simulink model "RRR_ADbst"  (R2022a)
settings: Solver=VariableStepAuto  StartTime=0.0  StopTime=500  RelTol=1e-6
undefined symbols (not defined in the file): DiscIntNeverNeededParam, dq0, Ks_ADbs, Lambda_ADbs, Levenberg, m1, m2, m3, Marquardt, p0, param, Pi, Pi_hat0_ADbs, q0, r0, r1, r2, R_ADbs, slow
libraries: simulink x1, robotmaniplib x1
settings Model: PauseTimes=0.14  Creator=Mathew  LastModifiedBy=Marco
settings SolverCC: ZeroCrossControl=DisableAll  ODENIntegrationMethod=ode1be
settings DebuggingCC: AlgebraicLoopMsg=none  UnconnectedInputMsg=warning  UnconnectedOutputMsg=warning  UnconnectedLineMsg=warning  SFMachineParentedDataDiag=warning
settings SFSimCC: CustomCodeUndefinedFunction=UseInterfaceOnly
settings RTWCC: DLArmComputeVersion=19.05

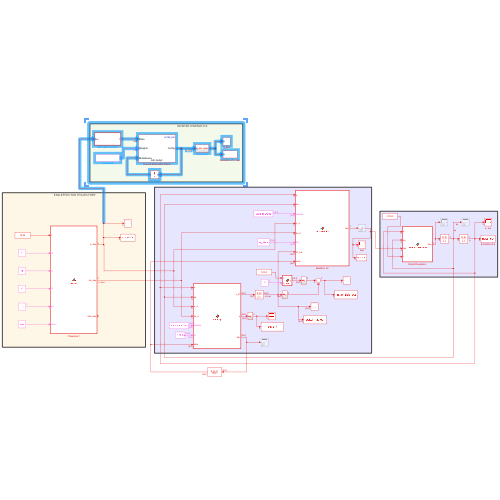
[thumbnail: Simulink's stored preview of the top-level diagram]
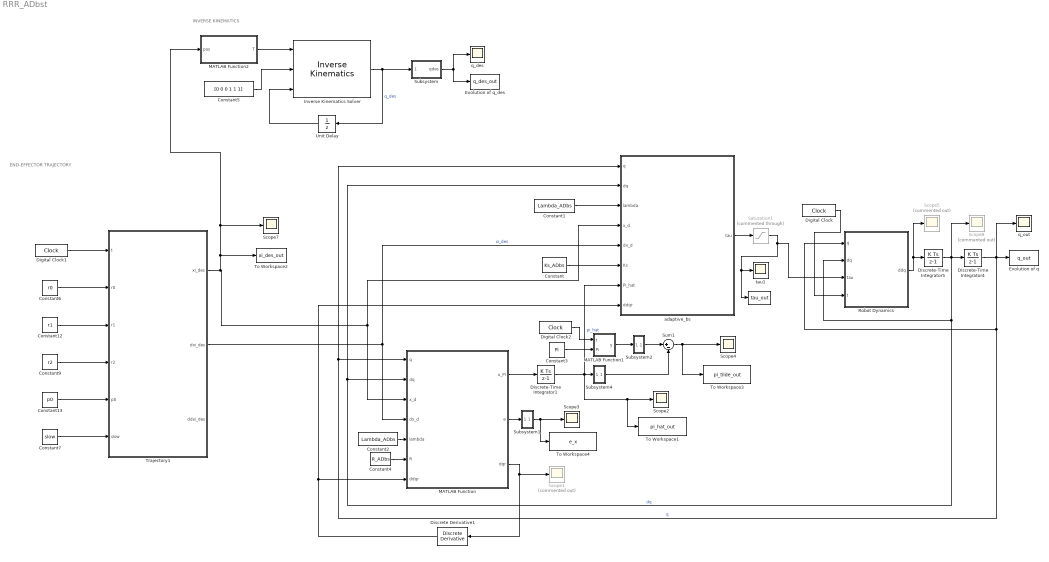
== system RRR_ADbst ==
  note: END-EFFECTOR TRAJECTORY
  note: INVERSE KINEMATICS
  "         " : ToWorkspace  VariableName=tau_out  SaveFormat=Timeseries  SampleTime=-1
  Constant : Constant  Value=Ks_ADbs
  Constant1 : Constant  Value=Lambda_ADbs
  Constant12 : Constant  Value=r1
  Constant13 : Constant  Value=p0
  Constant2 : Constant  Value=Lambda_ADbs
  Constant3 : Constant  Value=Pi
  Constant4 : Constant  Value=R_ADbs
  Constant5 : Constant  Value=[0 0 0 1 1 1]
  Constant6 : Constant  Value=r0
  Constant7 : Constant  Value=slow
  Constant9 : Constant  Value=r2
  Digital Clock : DigitalClock  SampleTime=0.01
  Digital Clock1 : DigitalClock  SampleTime=0.01
  Digital Clock2 : DigitalClock  SampleTime=0.01
  Discrete Derivative1 : simulink/Discrete/Discrete Derivative  gainval=1.0  ICPrevScaledInput=ddq0  OutMin=[]  OutMax=[]  OutDataType=fixdt(1, 16)  OutScaling=2^-10  DoSatur=off
  Discrete-Time Integrator1 : DiscreteIntegrator  InitialCondition=Pi_hat0_ADbs  SampleTime=-1  ICPrevOutput=DiscIntNeverNeededParam  ICPrevScaledInput=DiscIntNeverNeededParam
  Discrete-Time Integrator4 : DiscreteIntegrator  InitialCondition=q0  SampleTime=-1  ICPrevOutput=DiscIntNeverNeededParam  ICPrevScaledInput=DiscIntNeverNeededParam
  Discrete-Time Integrator5 : DiscreteIntegrator  InitialCondition=dq0  SampleTime=-1  ICPrevOutput=DiscIntNeverNeededParam  ICPrevScaledInput=DiscIntNeverNeededParam
  Evolution of q : ToWorkspace  VariableName=q_out  SaveFormat=Timeseries  SampleTime=-1
  Evolution of q_des : ToWorkspace  VariableName=q_des_out  SaveFormat=Timeseries  SampleTime=-1
  Inverse Kinematics Solver : robotmaniplib/Inverse Kinematics  RigidBodyTree=ur10e_bis  EndEffector=body3  ShowInfo=off  SolverName=Levenberg-Marquardt  EnforceJointLimits=on  MaxIterations=1500  MaxTime=10  GradientTolerance=1e-7  SolutionTolerance=1e-5  StepTolerance=1e-14  ErrorChangeTolerance=1e-8  UseErrorDamping=on  DampingBias=0.0025  SimulateUsing=Interpreted execution
  MATLAB Function : MATLAB Function  TreatAsAtomicUnit=on
  MATLAB Function1 : MATLAB Function  TreatAsAtomicUnit=on
  MATLAB Function2 : MATLAB Function  TreatAsAtomicUnit=on
  Robot Dynamics : MATLAB Function  TreatAsAtomicUnit=on
  Saturation1 : Saturate  Commented=through  UpperLimit=100  LowerLimit=-100
  Scope1 : Scope  Commented=on
  Scope{2..4,7} (4 alike) : Scope
  Scope5 : Scope  Commented=on
  Scope8 : Scope  Commented=on
  Subsystem : Subsystem
  Subsystem1 : Subsystem
  Subsystem2 : Subsystem
  Subsystem4 : Subsystem
  Sum1 : Sum  Inputs=|+-
  To Workspace1 : ToWorkspace  VariableName=pi_hat_out  SaveFormat=Timeseries  SampleTime=-1
  To Workspace2 : ToWorkspace  VariableName=xi_des_out  SaveFormat=Timeseries  SampleTime=-1
  To Workspace3 : ToWorkspace  VariableName=pi_tilde_out  SaveFormat=Timeseries  SampleTime=-1
  To Workspace4 : ToWorkspace  VariableName=e_x  SaveFormat=Timeseries  SampleTime=-1
  Trajectory1 : MATLAB Function  TreatAsAtomicUnit=on
  Unit Delay : UnitDelay  SampleTime=-1  HasFrameUpgradeWarning=on
  adaptive_bs : MATLAB Function  TreatAsAtomicUnit=on
  q_des : Scope
  q_out : Scope
  tau1 : Scope
  wires:
  Constant/1 -> adaptive_bs/6(Ks)
  adaptive_bs/1(tau) -> Saturation1/1
  MATLAB Function/1(u_Pi) -> Discrete-Time Integrator1/1
  Sum1/1 -> To Workspace3/1, Scope4/1
  Discrete-Time Integrator1/1 -> To Workspace1/1, Scope2/1, Subsystem4/1(eq), adaptive_bs/7(Pi_hat)  "pi_hat"
  Constant4/1 -> MATLAB Function/6(R)
  Constant2/1 -> MATLAB Function/5(lambda)
  Constant1/1 -> adaptive_bs/3(lambda)
  MATLAB Function/3(dqr) -> Discrete Derivative1/1, Scope1/1
  MATLAB Function/2(e) -> Subsystem1/1(eq)
  Digital Clock/1 -> Robot Dynamics/4(t)
  Discrete-Time Integrator5/1 -> Scope8/1, adaptive_bs/2(dq), MATLAB Function/2(dq), Robot Dynamics/2(dq), Discrete-Time Integrator4/1  "dq"
  Discrete-Time Integrator4/1 -> Evolution of q/1, adaptive_bs/1(q), MATLAB Function/1(q), Robot Dynamics/1(q), q_out/1  "q"
  Robot Dynamics/1(ddq) -> Scope5/1, Discrete-Time Integrator5/1
  Inverse Kinematics Solver/1 -> Subsystem/1(q_des), Unit Delay/1  "q_des"
  Subsystem/1(qdes) -> Evolution of q_des/1, q_des/1
  Saturation1/1 -> "         "/1, tau1/1, Robot Dynamics/3(tau)
  Trajectory1/1(xi_des) -> adaptive_bs/4(x_d), MATLAB Function/3(x_d), MATLAB Function2/1(pos), Scope7/1, To Workspace2/1
  Subsystem4/1(eq_) -> Sum1/2
  Subsystem1/1(eq_) -> To Workspace4/1, Scope3/1
  Trajectory1/2(dxi_des) -> adaptive_bs/5(dx_d), MATLAB Function/4(dx_d)  "xi_des"
  Constant13/1 -> Trajectory1/5(p0)
  Constant7/1 -> Trajectory1/6(slow)
  Constant9/1 -> Trajectory1/4(r2)
  Constant12/1 -> Trajectory1/3(r1)
  Constant5/1 -> Inverse Kinematics Solver/2
  MATLAB Function2/1(T) -> Inverse Kinematics Solver/1
  Unit Delay/1 -> Inverse Kinematics Solver/3
  Digital Clock1/1 -> Trajectory1/1(t)
  Constant6/1 -> Trajectory1/2(r0)
  MATLAB Function1/1(y) -> Subsystem2/1(eq)
  Constant3/1 -> MATLAB Function1/2(Pi)
  Digital Clock2/1 -> MATLAB Function1/1(t)
  Subsystem2/1(eq_) -> Sum1/1
  Discrete Derivative1/1 -> MATLAB Function/7(ddqr), adaptive_bs/8(ddqr)

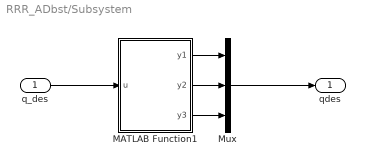
== system RRR_ADbst/Subsystem ==
  q_des : Inport
  MATLAB Function1 : MATLAB Function  TreatAsAtomicUnit=on
  Mux : Mux  Inputs=3
  qdes : Outport
  wires:
  MATLAB Function1/3(y3) -> Mux/3
  MATLAB Function1/2(y2) -> Mux/2
  q_des/1 -> MATLAB Function1/1(u)
  Mux/1 -> qdes/1
  MATLAB Function1/1(y1) -> Mux/1

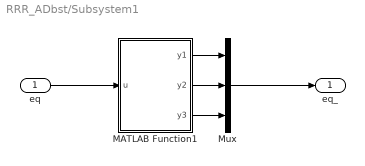
== system RRR_ADbst/Subsystem1 ==
  eq : Inport
  MATLAB Function1 : MATLAB Function  TreatAsAtomicUnit=on
  Mux : Mux  Inputs=3
  eq_ : Outport
  wires:
  MATLAB Function1/3(y3) -> Mux/3
  MATLAB Function1/2(y2) -> Mux/2
  eq/1 -> MATLAB Function1/1(u)
  Mux/1 -> eq_/1
  MATLAB Function1/1(y1) -> Mux/1

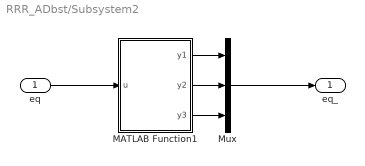
== system RRR_ADbst/Subsystem2 ==
  eq : Inport
  MATLAB Function1 : MATLAB Function  TreatAsAtomicUnit=on
  Mux : Mux  Inputs=3
  eq_ : Outport
  wires:
  MATLAB Function1/1(y1) -> Mux/1
  Mux/1 -> eq_/1
  eq/1 -> MATLAB Function1/1(u)
  MATLAB Function1/2(y2) -> Mux/2
  MATLAB Function1/3(y3) -> Mux/3

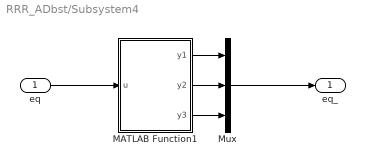
== system RRR_ADbst/Subsystem4 ==
  eq : Inport
  MATLAB Function1 : MATLAB Function  TreatAsAtomicUnit=on
  Mux : Mux  Inputs=3
  eq_ : Outport
  wires:
  MATLAB Function1/1(y1) -> Mux/1
  Mux/1 -> eq_/1
  eq/1 -> MATLAB Function1/1(u)
  MATLAB Function1/2(y2) -> Mux/2
  MATLAB Function1/3(y3) -> Mux/3

== matlab function RRR_ADbst/MATLAB Function1 ==
  data: t input; Pi input; y output
function y = fcn(t,Pi)

    if t > 200
        Pi(2) = Pi(2) + 1;
    end

    y = Pi;

end

== matlab function RRR_ADbst/Subsystem2/MATLAB Function1 ==
  data: u input; y1 output; y2 output; y3 output
function [y1,y2,y3] = fcn(u)

y1 = squeeze(u(1));
y2 = squeeze(u(2));
y3 = squeeze(u(3));

== matlab function RRR_ADbst/Subsystem4/MATLAB Function1 ==
  data: u input; y1 output; y2 output; y3 output
function [y1,y2,y3] = fcn(u)

y1 = squeeze(u(1));
y2 = squeeze(u(2));
y3 = squeeze(u(3));

== matlab function RRR_ADbst/MATLAB Function2 ==
  data: pos input; T output
function T = homogeneus_transf(pos)
    
    T=eye(4);
    
    T = [  eye(3),     [pos(1);pos(2);pos(3) ];
         0 0 0              1           ]; 

end

== matlab function RRR_ADbst/MATLAB Function ==
  data: q input; u_Pi output; dq input; x_d input; dx_d input; param parameter; lambda input; R input; e output; dqr output; ddqr input
function [u_Pi,e,dqr] = updating(q, dq, x_d, dx_d, param, lambda, R,ddqr)

    g = 9.81;
  
    RR = FK_3r(param,q);
    x = RR(1:3,4);
    
    J = J_3r(param,q);
    J = J(1:3,:);

    e  = x_d - x;
    dqr = pinv(J) * (dx_d + lambda * e);

    s = dqr - dq;
    
    Y = Y_fun_SL(g,param,ddqr,dqr,dq,q);
    
    u_Pi = pinv(R) * Y' * s;
    
end

== matlab function RRR_ADbst/Subsystem1/MATLAB Function1 ==
  data: u input; y1 output; y2 output; y3 output
function [y1,y2,y3] = fcn(u)

y1 = squeeze(u(1));
y2 = squeeze(u(2));
y3 = squeeze(u(3));

== matlab function RRR_ADbst/Robot Dynamics ==
  data: q input; dq input; tau input; t input; ddq output; m1 parameter; m2 parameter; m3 parameter; param parameter
function ddq = inverse_dynamics(q, dq, tau, t, m1, m2, m3, param)
    
    g = 9.81;

    if t > 200
        m2 = m2 + 1;
    end

    % Get dynamic matrices
    M = B_3r(param,m1,m2,m3,q);
    C = C_3r(param,m1,m2,m3,q,dq);
    G = G_3r(g,param,m1,m2,m3,q);
    
    ddq = pinv(M)*(tau - C*dq - G);

end

== matlab function RRR_ADbst/Subsystem/MATLAB Function1 ==
  data: u input; y1 output; y2 output; y3 output
function [y1,y2,y3] = fcn(u)

y1 = squeeze(u(1));
y2 = squeeze(u(2));
y3 = squeeze(u(3));

== matlab function RRR_ADbst/adaptive_bs ==
  data: q input; dq input; lambda input; x_d input; dx_d input; tau output; Ks input; Pi_hat input; param parameter; ddqr input
function tau = adaptive_bs(q, dq, lambda, x_d, dx_d, Ks, Pi_hat, param,ddqr)
    
    g = 9.81;
  
    RR = FK_3r(param,q);
    x = RR(1:3,4);
    
    J = J_3r(param,q);
    J = J(1:3,:);
    
    e  = x_d - x;
    dqr = pinv(J) * (dx_d + lambda * e);                                        
    
    s = dqr - dq;
    
    Y = Y_fun_SL(g,param,ddqr,dqr,dq,q);

    % Control law
    tau = Y*Pi_hat + Ks*s + J' * e;

end

== matlab function RRR_ADbst/Trajectory1 ==
  data: t input; r0 input; xi_des output; r1 input; r2 input; p0 input; slow input; dxi_des output; ddxi_des output
function [xi_des, dxi_des, ddxi_des] = trajectory(t,r0,r1,r2,p0,slow)

    k=slow;
    
    xi_des =   [r0*sin(t/(2*k))       ; r1*sin(t/k)     ; r2*cos(t/k)     ] + p0;
    dxi_des =  [r0/2/k*cos(t/(2*k))   ; r1/k*cos(t/k)   ; -r2/k*sin(t/k)  ];
    ddxi_des = [-r0/4/k/k*sin(t/(2*k)); -r1/k/k*sin(t/k); -r2/k/k*cos(t/k)];

end
